simulink model "vC_3ph_MR2"  (Simulink 7.9)
settings: Solver=ode14x  StartTime=0.0  StopTime=20/60  FixedStep=Ts1  RelTol=1e-3
PostLoadFcn:
  | , if any(exist('dsrtsu_mdlpostloadfcn', 'file') == [2, 3, 6]), try dsrtsu_mdlpostloadfcn('Execute', bdroot); catch fprintf('Error in PostLoadFcn (dsrtsu_mdlpostloadfcn) for model "%s":\n %s\n', bdroot, lasterr); end, end,
InitFcn:
  | vC_ini
values from neighbouring files (symbols this model uses):
  C = Cideal+deltaC    (= 4e-05)    [IMC_calculo_limites_thetas.m]    (also in IMC_ini.m; JORGE_controlador_LCL_malha_interna.m; LCL_PAPM.m; R_in_LCL.m)
  excitacao_persistente = 0    [iC_ini.m]    (also in vC_ini.m)
  flag_time = 60/60    (= 1)    [iC_ini.m]    (also in vC_ini.m = 0)
  init_time = 60/60    (= 1)    [iC_ini.m]    (also in vC_ini.m)
  L1 = L1ideal+deltaL1    (= 0.002)    [IMC_calculo_limites_thetas.m]    (also in IMC_ini.m; LCL_PAPM.m; R_in_LCL.m; calculo_FTs.m)
  L2 = L2ideal+deltaL2+Lgideal+deltaLg    (= 0.002)    [IMC_calculo_limites_thetas.m]    (also in IMC_ini.m; LCL_PAPM.m; R_in_LCL.m; calculo_FTs.m)
  param_change_time = 60/60    (= 1)    [iC_ini.m]    (also in vC_ini.m)
  R1 = R1ideal+deltaR1    (= 1)    [IMC_calculo_limites_thetas.m]    (also in IMC_ini.m; R_in_LCL.m = 0; gera_resultados.m = 0; iC_ini.m = 0)
  R2 = R2ideal+deltaR2+Rgideal+deltaRg    (= 1)    [IMC_calculo_limites_thetas.m]    (also in IMC_ini.m; R_in_LCL.m = 0; gera_resultados.m = 0; iC_ini.m = 0)
  R_init = 10    [iC_ini.m]    (also in vC_ini.m)
  ref_phaseInv_time = 60/60    (= 1)    [iC_ini.m]    (also in vC_ini.m)
  ref_step_time = 60/60    (= 1)    [iC_ini.m]    (also in vC_ini.m)
  short_OFF_time = 61/60    (= 1.01666666667)    [vC_ini.m]
  short_ON_time = 60/60    (= 1)    [vC_ini.m]
  Ts = 0.5    [IMC_calculo_limites_thetas.m]    (also in IMC_datta_ini.m; IMC_ini.m = 8.33333333333e-05; JORGE_controlador_LCL_malha_interna.m = 8.33333333333e-05; LCL_PAPM.m = 8.33333333333e-05)
  Ts1 = Ts/10    (= 8.33333333333e-06)    [iC_ini.m]    (also in vC_ini.m)
  VCC = 1700    [iC_ini.m]    (also in vC_ini.m = 1200)
undefined symbols (not defined in the file or in its folder): D1, Delta
libraries: powerlib x38, powerlib_extras x1
(part 2 of 3)

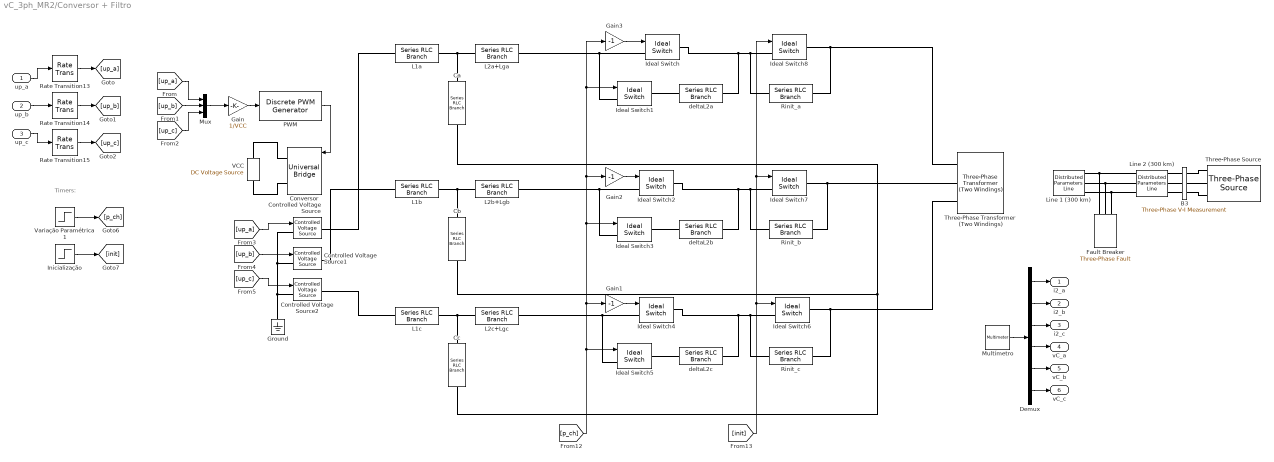
== system vC_3ph_MR2/Conversor + Filtro ==
  note: Timers:
  up_a : Inport
  up_b : Inport  Port=2
  up_c : Inport  Port=3
  B3 : powerlib/Measurements/Three-Phase V-I Measurement  VoltageMeasurement=no  SetLabelV=on  LabelV=Vabc_B3  Vpu=on  VpuLL=off  CurrentMeasurement=no  SetLabelI=on  LabelI=Iabc_B3  Ipu=on  Pbase=100e6  Vbase=735e3  OutputType=Complex  PhasorSimulation=off  PSBequivalent=0
  Ca : powerlib/Elements/Series RLC Branch  LConnTagsString=__new0  RConnTagsString=__new0  BranchType=C  Resistance=1  Inductance=1e-3  SetiL0=off  InitialCurrent=0  Capacitance=C  Setx0=off  InitialVoltage=0  Measurements=Branch voltage
  Cb : powerlib/Elements/Series RLC Branch  LConnTagsString=__new0  RConnTagsString=__new0  BranchType=C  Resistance=1  Inductance=1e-3  SetiL0=off  InitialCurrent=0  Capacitance=C  Setx0=off  InitialVoltage=0  Measurements=Branch voltage
  Cc : powerlib/Elements/Series RLC Branch  LConnTagsString=__new0  RConnTagsString=__new0  BranchType=C  Resistance=1  Inductance=1e-3  SetiL0=off  InitialCurrent=0  Capacitance=C  Setx0=off  InitialVoltage=0  Measurements=Branch voltage
  Controlled Voltage Source : powerlib/Electrical Sources/Controlled Voltage Source  Initialize=on  Source_Type=AC  Amplitude=0  Phase=0  Frequency=0  Measurements=None
  Controlled Voltage Source1 : powerlib/Electrical Sources/Controlled Voltage Source  Initialize=on  Source_Type=AC  Amplitude=0  Phase=0  Frequency=0  Measurements=None
  Controlled Voltage Source2 : powerlib/Electrical Sources/Controlled Voltage Source  Initialize=on  Source_Type=AC  Amplitude=0  Phase=0  Frequency=0  Measurements=None
  Conversor : powerlib/Power Electronics/Universal Bridge  Arms=3  SnubberResistance=1e5  SnubberCapacitance=inf  Device=IGBT / Diodes  Ron=1e-3  Lon=0  ForwardVoltages="[  0  0  ]"  ForwardVoltage=0  GTOparameters=[ 10e-6 , 20e-6 ]  IGBTparameters=[ 1e-6 , 2e-6 ]  Measurements=UAB UBC UCA UDC voltages  Measurements_2=None  converterType=Rectifier
  Demux : Demux  Outputs=6
  Fault Breaker : powerlib/Elements/Three-Phase Fault  FaultA=on  FaultB=off  FaultC=off  FaultResistance=0.001  GroundFault=on  GroundResistance=1  External=off  SwitchStatus=[1 0]  SwitchTimes=[ short_ON_time short_OFF_time ]  InitialStates=[0 0 1]  SnubberResistance=inf  SnubberCapacitance=inf  Measurements=Fault currents
  Gain : Gain  Gain=1/VCC  SampleTime=Ts1
  Gain1 : Gain  Gain=-1  SampleTime=Ts1
  Gain2 : Gain  Gain=-1  SampleTime=Ts1
  Gain3 : Gain  Gain=-1  SampleTime=Ts1
  Ground : powerlib/Elements/Ground  LConnTagsString=a
  Ideal Switch : powerlib/Power Electronics/Ideal Switch  Ron=0.001  Lon=0  IC=1  Rs=1e5  Cs=inf  Measurements=off
  Ideal Switch{1,3,5..8} (6 alike) : powerlib/Power Electronics/Ideal Switch  Ron=0.001  Lon=0  IC=0  Rs=1e5  Cs=inf  Measurements=off
  Ideal Switch2 : powerlib/Power Electronics/Ideal Switch  Ron=0.001  Lon=0  IC=1  Rs=1e5  Cs=inf  Measurements=off
  Ideal Switch4 : powerlib/Power Electronics/Ideal Switch  Ron=0.001  Lon=0  IC=1  Rs=1e5  Cs=inf  Measurements=off
  Inicialização : Step  Time=init_time  SampleTime=Ts1
  L1a : powerlib/Elements/Series RLC Branch  LConnTagsString=__new0  RConnTagsString=__new0  BranchType=RL  Resistance=R1  Inductance=L1  SetiL0=off  InitialCurrent=0  Capacitance=1e-6  Setx0=off  InitialVoltage=0  Measurements=None
  L1b : powerlib/Elements/Series RLC Branch  LConnTagsString=__new0  RConnTagsString=__new0  BranchType=RL  Resistance=R1  Inductance=L1  SetiL0=off  InitialCurrent=0  Capacitance=1e-6  Setx0=off  InitialVoltage=0  Measurements=None
  L1c : powerlib/Elements/Series RLC Branch  LConnTagsString=__new0  RConnTagsString=__new0  BranchType=RL  Resistance=R1  Inductance=L1  SetiL0=off  InitialCurrent=0  Capacitance=1e-6  Setx0=off  InitialVoltage=0  Measurements=None
  L2a+Lga : powerlib/Elements/Series RLC Branch  LConnTagsString=__new0  RConnTagsString=__new0  BranchType=RL  Resistance=R2  Inductance=L2  SetiL0=off  InitialCurrent=0  Capacitance=1e-6  Setx0=off  InitialVoltage=0  Measurements=Branch current
  L2b+Lgb : powerlib/Elements/Series RLC Branch  LConnTagsString=__new0  RConnTagsString=__new0  BranchType=RL  Resistance=R2  Inductance=L2  SetiL0=off  InitialCurrent=0  Capacitance=1e-6  Setx0=off  InitialVoltage=0  Measurements=Branch current
  L2c+Lgc : powerlib/Elements/Series RLC Branch  LConnTagsString=__new0  RConnTagsString=__new0  BranchType=RL  Resistance=R2  Inductance=L2  SetiL0=off  InitialCurrent=0  Capacitance=1e-6  Setx0=off  InitialVoltage=0  Measurements=Branch current
  Line 1 (300 km) : powerlib/Elements/Distributed Parameters Line  Phases=3  Frequency=60  Resistance=[0.01273 0.3864]  Inductance="[0.9337e-3  4.1264e-3]"  Capacitance=[12.74e-9 7.751e-9]  Length=300  x1=[-0.0017 3.92005703085229e-11 -7396.02996094138 -52768.9690973413;-0.00169166666666667 3.90926214322584e-11 -7230.2151300675 -52791.9439683011;-0.00168333333333333 3.89842867276027e-11 -7064.32893988924 -52814.3978040869;-0.001675 3.88755672637756e-11 -6898.37302763633 -52836.3303830885;-0.00166666666666667 3.87664641137943e-11 -6732.34903122663 -52857.74148884;-0.00165833333333333 3.86569783544628e-11 -6566.25858924993 -52878.6309100226;-0.00165 3.85471110663615e-11 -6400.10334095188 -52898.9984404661;-0.00164166666666667 3.8436863333836e-11 -6233.88492621767 -52918.8438791512;-0.00163333333333333 3.8326236244987e-11 -6067.60498555597 -52938.1670302113;-0.001625 3.82152308916592e-11 -5901.26516008265 -52956.9677029349;-0.00161666666666667 3.81038483694306e-11 -5734.86709150463 -52975.2457117669;-0.00160833333333333 3.79920897776017e-11 -5568.41242210368 -52993.0008763106;-0.0016 3.78799562191848e-11 -5401.90279472019 -53010.2330213299;-0.00159166666666667 3.77674488008927e-11 -5235.33985273694 -53026.9419767503;-0.00158333333333333 3.76545686331283e-11 -5068.72524006294 -53043.1275776612;-0.001575 3.75413168299733e-11 -4902.06060111715 -53058.7896643174;-0.00156666666666667 3.74276945091772e-11 -4735.34758081227 -53073.9280821402;-0.00155833333333333 3.73137027921465e-11 -4568.5878245385 -53088.5426817197;-0.00155 3.71993428039333e-11 -4401.78297814733 -53102.6333188156;-0.00154166666666667 3.70846156732247e-11 -4234.93468793522 -53116.1998543591;-0.00153333333333333 3.6969522532331e-11 -4068.04460062746 -53129.2421544539;-0.001525 3.68540645171751e-11 -3901.11436336182 -53141.7600903778;-0.00151666666666667 3.67382427672811e-11 -3734.14562367236 -53153.7535385837;-0.00150833333333333 3.66220584257627e-11 -3567.14002947314 -53165.2223807013;-0.0015 3.65055126393127e-11 -3400.09922904194 -53176.1665035377;-0.00149166666666667 3.63886065581907e-11 -3233.02487100401 -53186.5857990787;-0.00148333333333333 3.62713413362127e-11 -3065.91860431584 -53196.4801644903;-0.001475 3.6153718130739e-11 -2898.78207824881 -53205.8495021188;-0.00146666666666667 3.60357381026632e-11 -2731.61694237295 -53214.6937194929;-0.00145833333333333 3.59174024164006e-11 -2564.42484654066 -53223.0127293236;-0.00145 3.57987122398765e-11 -2397.20744087044 -53230.8064495056;-0.00144166666666667 3.56796687445152e-11 -2229.96637573058 -53238.0748031182;-0.00143333333333333 3.55602731052279e-11 -2062.70330172285 -53244.8177184255;-0.001425 3.54405265004012e-11 -1895.41986966628 -53251.0351288777;-0.00141666666666667 3.53204301118859e-11 -1728.11773058082 -53256.7269731115;-0.00140833333333333 3.51999851249848e-11 -1560.79853567102 -53261.8931949508;-0.0014 3.50791927284414e-11 -1393.46393630979 -53266.5337434068;-0.00139166666666667 3.49580541144278e-11 -1226.11558402208 -53270.6485726794;-0.00138333333333333 3.48365704785332e-11 -1058.75513046855 -53274.2376421568;-0.001375 3.47147430197521e-11 -891.384227429335 -53277.3009164164;-0.00136666666666667 3.45925729404722e-11 -724.004526787645 -53279.8383652248;-0.00135833333333333 3.44700614464631e-11 -556.617680513576 -53281.8499635386;-0.00135 3.43472097468636e-11 -389.225340647714 -53283.3356915039;-0.00134166666666667 3.42240190541704e-11 -221.82915928488 -53284.2955344573;-0.00133333333333333 3.41004905842259e-11 -54.4307885578019 -53284.7294829255;-0.001325 3.39766255562063e-11 112.968119379191 -53284.6375326256;-0.00131666666666667 3.38524251926094e-11 280.365912366451 -53284.0196844652;-0.00130833333333333 3.37278907192426e-11 447.760938255349 -53282.8759445421;-0.0013 3.3603023365211e-11 615.151544924549 -53281.2063241446;-0.00129166666666667 3.34778243629047e-11 782.536080296351 -53279.0108397512;-0.00128333333333333 3.33522949479876e-11 949.912892352961 -53276.2895130304;-0.001275 3.32264363593842e-11 1117.28032915281 -53273.0423708406;-0.00126666666666667 3.3100249839268e-11 1284.63673884689 -53269.2694452298;-0.00125833333333333 3.2973736633049e-11 1451.98046969498 -53264.9707734353;-0.00125 ...(+10984 chars)]  x2=[-0.0017 -3.86024177087245e-11 -6618.00740677682 -48900.0765944437;-0.00169166666666667 -3.86499120226598e-11 -6464.35087955851 -48920.6263316872;-0.00168333333333333 -3.8697024877567e-11 -6310.63055180679 -48940.6932420988;-0.001675 -3.87437558084613e-11 -6156.84794067921 -48960.2771276263;-0.00166666666666667 -3.87901043541273e-11 -6003.0045639481 -48979.3777949846;-0.00165833333333333 -3.88360700571234e-11 -5849.10193998543 -48997.9950556579;-0.00165 -3.88816524637869e-11 -5695.14158774801 -49016.1287259012;-0.00164166666666667 -3.89268511242377e-11 -5541.12502676233 -49033.7786267426;-0.00163333333333333 -3.89716655923833e-11 -5387.05377710968 -49050.9445839847;-0.001625 -3.9016095425923e-11 -5232.92935941109 -49067.6264282065;-0.00161666666666667 -3.90601401863523e-11 -5078.75329481235 -49083.8239947648;-0.00160833333333333 -3.91037994389672e-11 -4924.52710496895 -49099.5371237962;-0.0016 -3.91470727528684e-11 -4770.25231203115 -49114.7656602185;-0.00159166666666667 -3.91899597009659e-11 -4615.93043862886 -49129.5094537321;-0.00158333333333333 -3.92324598599828e-11 -4461.56300785665 -49143.7683588218;-0.001575 -3.92745728104597e-11 -4307.15154325877 -49157.542234758;-0.00156666666666667 -3.93162981367586e-11 -4152.69756881403 -49170.830945598;-0.00155833333333333 -3.93576354270677e-11 -3998.20260892079 -49183.6343601876;-0.00155 -3.93985842734043e-11 -3843.66818838195 -49195.9523521624;-0.00154166666666667 -3.94391442716201e-11 -3689.09583238984 -49207.7847999486;-0.00153333333333333 -3.94793150214041e-11 -3534.48706651121 -49219.1315867649;-0.001525 -3.95190961262872e-11 -3379.84341667215 -49229.9926006229;-0.00151666666666667 -3.95584871936462e-11 -3225.16640914308 -49240.367734329;-0.00150833333333333 -3.95974878347069e-11 -3070.4575705236 -49250.2568854846;-0.0015 -3.96360976645489e-11 -2915.7184277275 -49259.6599564879;-0.00149166666666667 -3.96743163021086e-11 -2760.95050796763 -49268.5768545344;-0.00148333333333333 -3.97121433701836e-11 -2606.15533874089 -49277.0074916179;-0.001475 -3.9749578495436e-11 -2451.33444781311 -49284.9517845313;-0.00146666666666667 -3.97866213083962e-11 -2296.48936320397 -49292.4096548678;-0.00145833333333333 -3.98232714434666e-11 -2141.62161317194 -49299.3810290211;-0.00145 -3.98595285389251e-11 -1986.73272619921 -49305.8658381866;-0.00144166666666667 -3.98953922369289e-11 -1831.82423097654 -49311.8640183619;-0.00143333333333333 -3.99308621835178e-11 -1676.89765638824 -49317.3755103474;-0.001425 -3.99659380286176e-11 -1521.95453149707 -49322.4002597467;-0.00141666666666667 -4.0000619426044e-11 -1366.99638552912 -49326.9382169678;-0.00140833333333333 -4.00349060335056e-11 -1212.02474785872 -49330.9893372228;-0.0014 -4.00687975126074e-11 -1057.04114799336 -49334.5535805287;-0.00139166666666667 -4.01022935288541e-11 -902.047115558624 -49337.630911708;-0.00138333333333333 -4.01353937516537e-11 -747.044180283028 -49340.2213003885;-0.001375 -4.01680978543202e-11 -592.033871982974 -49342.3247210043;-0.00136666666666667 -4.02004055140775e-11 -437.017720547603 -49343.9411527954;-0.00135833333333333 -4.02323164120619e-11 -281.997255923769 -49345.0705798083;-0.00135 -4.02638302333257e-11 -126.97400810086 -49345.7129908959;-0.00134166666666667 -4.02949466668403e-11 28.0504929042399 -49345.868379718;-0.00133333333333333 -4.0325665405499e-11 183.0747170623 -49345.536744741;-0.001325 -4.03559861461203e-11 338.097134346815 -49344.7180892378;-0.00131666666666667 -4.03859085894508e-11 493.116214749112 -49343.4124212884;-0.00130833333333333 -4.04154324401678e-11 648.130428293447 -49341.6197537792;-0.0013 -4.04445574068831e-11 803.138245052112 -49339.3401044029;-0.00129166666666667 -4.04732832021449e-11 958.138135160545 -49336.573495659;-0.00128333333333333 -4.05016095424412e-11 1113.1285688324 -49333.3199548526;-0.001275 -4.05295361482025e-11 1268.10801637466 -49329.5795140949;-0.00126666666666667 -4.05570627438045e-11 1423.07494820276 -49325.3522103026;-0.00125833333333333 -4.05841890575707e-11 ...(+11172 chars)]  x3=[-0.0017 -2.15563861094982e-14 -27.7294039862374 -193.67611553396;-0.00169166666666667 -2.22240906952308e-14 -27.1208166863509 -193.762274129979;-0.00168333333333333 -2.28915759381605e-14 -26.5119617149528 -193.846520370577;-0.001675 -2.35588352504773e-14 -25.9028450811959 -193.928853424279;-0.00166666666666667 -2.42258620466013e-14 -25.2934727968154 -194.009272478489;-0.00165833333333333 -2.48926497432473e-14 -24.6838508760698 -194.087776739504;-0.00165 -2.55591917594899e-14 -24.0739853356814 -194.16436543252;-0.00164166666666667 -2.62254815168285e-14 -23.4638821947767 -194.239037801636;-0.00163333333333333 -2.68915124392521e-14 -22.8535474748276 -194.311793109867;-0.001625 -2.75572779533045e-14 -22.2429871995912 -194.382630639146;-0.00161666666666667 -2.82227714881489e-14 -21.632207395051 -194.451549690336;-0.00160833333333333 -2.88879864756327e-14 -21.021214089357 -194.518549583234;-0.0016 -2.95529163503525e-14 -20.4100133127667 -194.583629656578;-0.00159166666666667 -3.02175545497189e-14 -19.7986110975848 -194.646789268054;-0.00158333333333333 -3.08818945140212e-14 -19.1870134781044 -194.708027794302;-0.001575 -3.15459296864923e-14 -18.575226490547 -194.767344630923;-0.00156666666666667 -3.22096535133728e-14 -17.9632561730033 -194.824739192482;-0.00155833333333333 -3.28730594439768e-14 -17.3511085653733 -194.88021091252;-0.00155 -3.35361409307555e-14 -16.7387897093067 -194.933759243553;-0.00154166666666667 -3.41988914293622e-14 -16.1263056481433 -194.985383657079;-0.00153333333333333 -3.48613043987172e-14 -15.5136624268536 -195.035083643588;-0.001525 -3.5523373301072e-14 -14.9008660919789 -195.08285871256;-0.00151666666666667 -3.61850916020735e-14 -14.2879226915716 -195.128708392475;-0.00150833333333333 -3.68464527708295e-14 -13.6748382751356 -195.172632230814;-0.0015 -3.75074502799721e-14 -13.0616188935666 -195.214629794068;-0.00149166666666667 -3.81680776057228e-14 -12.4482705990923 -195.254700667737;-0.00148333333333333 -3.88283282279567e-14 -11.8347994452128 -195.292844456338;-0.001475 -3.94881956302665e-14 -11.2212114866406 -195.329060783407;-0.00146666666666667 -4.01476733000276e-14 -10.6075127792412 -195.363349291503;-0.00145833333333333 -4.08067547284614e-14 -9.99370937997315 -195.395709642214;-0.00145 -4.14654334107004e-14 -9.37980734682814 -195.426141516155;-0.00144166666666667 -4.21237028458519e-14 -8.7658127387714 -195.454644612975;-0.00143333333333333 -4.27815565370624e-14 -8.15173161568181 -195.481218651362;-0.001425 -4.34389879915814e-14 -7.53757003829216 -195.50586336904;-0.00141666666666667 -4.4095990720826e-14 -6.92333406812929 -195.528578522775;-0.00140833333333333 -4.47525582404444e-14 -6.30902976745423 -195.549363888378;-0.0014 -4.54086840703804e-14 -5.69466319920241 -195.568219260705;-0.00139166666666667 -4.60643617349368e-14 -5.08024042692384 -195.585144453663;-0.00138333333333333 -4.67195847628398e-14 -4.46576751472323 -195.600139300206;-0.001375 -4.73743466873027e-14 -3.85125052720019 -195.613203652342;-0.00136666666666667 -4.80286410460896e-14 -3.23669552938921 -195.624337381129;-0.00135833333333333 -4.86824613815793e-14 -2.62210858670008 -195.633540376683;-0.00135 -4.9335801240829e-14 -2.00749576485779 -195.640812548174;-0.00134166666666667 -4.99886541756382e-14 -1.39286312984277 -195.646153823829;-0.00133333333333333 -5.06410137426119e-14 -0.778216747830982 -195.649564150931;-0.001325 -5.12928735032246e-14 -0.163562685134053 -195.651043495821;-0.00131666666666667 -5.19442270238835e-14 0.451092991860548 -195.6505918439;-0.00130833333333333 -5.25950678759925e-14 1.06574421674942 -195.648209199625;-0.0013 -5.3245389636015e-14 1.68038492317314 -195.643895586511;-0.00129166666666667 -5.38951858855379e-14 2.29500904487608 -195.637651047133;-0.00128333333333333 -5.45444502113344e-14 2.90961051576626 -195.62947564312;-0.001275 -5.51931762054278e-14 3.52418326997528 -195.619369455162;-0.00126666666666667 -5.58413574651545e-14 4.13872124191825 -195.607332583003;-0.00125833333333333 -5.6488987593227e-14 ...(+11158 chars)]  x4=[-0.0017 -1.25069855625768e-15 -97.1520132574429 -167.719905551199;-0.00169166666666667 -1.17646120080317e-15 -96.6246270754558 -168.024289436398;-0.00168333333333333 -1.10221223415156e-15 -96.0962872474085 -168.327014989695;-0.001675 -1.02795238911018e-15 -95.5669989878017 -168.62807922331;-0.00166666666666667 -9.53682398593721e-16 -95.0367675204968 -168.927479165861;-0.00165833333333333 -8.79402995617002e-16 -94.5055980786644 -169.225211862392;-0.00165 -8.05114913287751e-16 -93.9734959047324 -169.5212743744;-0.00164166666666667 -7.30818884799338e-16 -93.4404662503344 -169.815663779869;-0.00163333333333333 -6.56515643423579e-16 -92.906514376258 -170.108377173294;-0.001625 -5.82205922503465e-16 -92.3716455523927 -170.399411665711;-0.00161666666666667 -5.07890455445944e-16 -91.8358650576776 -170.688764384729;-0.00160833333333333 -4.33569975714665e-16 -91.29917818005 -170.976432474552;-0.0016 -3.59245216822771e-16 -90.7615902163928 -171.262413096012;-0.00159166666666667 -2.84916912325618e-16 -90.2231064724821 -171.546703426596;-0.00158333333333333 -2.10585795813567e-16 -89.6837322629351 -171.829300660474;-0.001575 -1.36252600904725e-16 -89.1434729111574 -172.110202008525;-0.00156666666666667 -6.19180612377231e-17 -88.6023337492907 -172.389404698365;-0.00155833333333333 1.24170895355471e-17 -88.0603201181601 -172.666905974378;-0.00155 8.67521177571522e-17 -87.5174373672214 -172.942703097737;-0.00154166666666667 1.61086289770384e-16 -86.9736908545081 -173.216793346436;-0.00153333333333333 2.35418871926968e-16 -86.4290859465787 -173.489174015315;-0.001525 3.09749130594331e-16 -85.8836280184639 -173.759842416088;-0.00151666666666667 3.84076332162822e-16 -85.3373224536132 -174.028795877365;-0.00150833333333333 4.58399743052972e-16 -84.7901746438419 -174.296031744685;-0.0015 5.32718629722723e-16 -84.2421899892781 -174.561547380538;-0.00149166666666667 6.07032258674666e-16 -83.693373898309 -174.825340164392;-0.00148333333333333 6.81339896463284e-16 -83.1437317875279 -175.087407492718;-0.001475 7.55640809702191e-16 -82.5932690816805 -175.347746779018;-0.00146666666666667 8.29934265071373e-16 -82.0419912136116 -175.606355453848;-0.00145833333333333 9.0421952932442e-16 -81.4899036242111 -175.863230964844;-0.00145 9.78495869295754e-16 -80.9370117623606 -176.11837077675;-0.00144166666666667 1.05276255190789e-15 -80.3833210848796 -176.371772371439;-0.00143333333333333 1.12701884417867e-15 -79.8288370564716 -176.623433247938;-0.001425 1.20126401322844e-15 -79.27356514967 -176.873350922457;-0.00141666666666667 1.27549732628738e-15 -78.7175108447845 -177.121522928408;-0.00140833333333333 1.34971805070264e-15 -78.1606796298464 -177.367946816436;-0.0014 1.42392545394565e-15 -77.6030770005551 -177.612620154434;-0.00139166666666667 1.49811880361929e-15 -77.0447084602235 -177.855540527577;-0.00138333333333333 1.57229736746515e-15 -76.4855795197236 -178.096705538338;-0.001375 1.64646041337075e-15 -75.9256956974323 -178.336112806516;-0.00136666666666667 1.72060720937678e-15 -75.3650625191769 -178.573759969258;-0.00135833333333333 1.79473702368429e-15 -74.8036855181805 -178.809644681081;-0.00135 1.86884912466194e-15 -74.2415702350076 -179.043764613901;-0.00134166666666667 1.94294278085322e-15 -73.6787222175089 -179.276117457046;-0.00133333333333333 2.01701726098364e-15 -73.1151470207673 -179.506700917289;-0.001325 2.09107183396801e-15 -72.5508502070424 -179.735512718863;-0.00131666666666667 2.16510576891757e-15 -71.9858373457159 -179.96255060349;-0.00130833333333333 2.23911833514728e-15 -71.4201140132366 -180.187812330395;-0.0013 2.31310880218299e-15 -70.8536857930655 -180.411295676338;-0.00129166666666667 2.38707643976867e-15 -70.2865582756204 -180.632998435627;-0.00128333333333333 2.46102051787358e-15 -69.718737058221 -180.852918420146;-0.001275 2.53494030669954e-15 -69.1502277450334 -181.071053459374;-0.00126666666666667 2.60883507668807e-15 -68.581035947015 -181.287401400405;-0.00125833333333333 2.68270409852762e-15 -68.0111672818591 ...(+11113 chars)]  x5=0.00169662470098723  Measurements=None
      settings: AttributesFormatString=\n
  Line 2 (300 km) : powerlib/Elements/Distributed Parameters Line  Phases=3  Frequency=60  Resistance=[0.01273 0.3864]  Inductance="[0.9337e-3  4.1264e-3]"  Capacitance=[12.74e-9 7.751e-9]  Length=300  x1=[-0.0017 -3.86024177087245e-11 -6618.00740677682 -48900.0765944437;-0.00169166666666667 -3.86499120226598e-11 -6464.35087955851 -48920.6263316872;-0.00168333333333333 -3.8697024877567e-11 -6310.63055180679 -48940.6932420988;-0.001675 -3.87437558084613e-11 -6156.84794067921 -48960.2771276263;-0.00166666666666667 -3.87901043541273e-11 -6003.0045639481 -48979.3777949846;-0.00165833333333333 -3.88360700571234e-11 -5849.10193998543 -48997.9950556579;-0.00165 -3.88816524637869e-11 -5695.14158774801 -49016.1287259012;-0.00164166666666667 -3.89268511242377e-11 -5541.12502676233 -49033.7786267426;-0.00163333333333333 -3.89716655923833e-11 -5387.05377710968 -49050.9445839847;-0.001625 -3.9016095425923e-11 -5232.92935941109 -49067.6264282065;-0.00161666666666667 -3.90601401863523e-11 -5078.75329481235 -49083.8239947648;-0.00160833333333333 -3.91037994389672e-11 -4924.52710496895 -49099.5371237962;-0.0016 -3.91470727528684e-11 -4770.25231203115 -49114.7656602185;-0.00159166666666667 -3.91899597009659e-11 -4615.93043862886 -49129.5094537321;-0.00158333333333333 -3.92324598599828e-11 -4461.56300785665 -49143.7683588218;-0.001575 -3.92745728104597e-11 -4307.15154325877 -49157.542234758;-0.00156666666666667 -3.93162981367586e-11 -4152.69756881403 -49170.830945598;-0.00155833333333333 -3.93576354270677e-11 -3998.20260892079 -49183.6343601876;-0.00155 -3.93985842734043e-11 -3843.66818838195 -49195.9523521624;-0.00154166666666667 -3.94391442716201e-11 -3689.09583238984 -49207.7847999486;-0.00153333333333333 -3.94793150214041e-11 -3534.48706651121 -49219.1315867649;-0.001525 -3.95190961262872e-11 -3379.84341667215 -49229.9926006229;-0.00151666666666667 -3.95584871936462e-11 -3225.16640914308 -49240.367734329;-0.00150833333333333 -3.95974878347069e-11 -3070.4575705236 -49250.2568854846;-0.0015 -3.96360976645489e-11 -2915.7184277275 -49259.6599564879;-0.00149166666666667 -3.96743163021086e-11 -2760.95050796763 -49268.5768545344;-0.00148333333333333 -3.97121433701836e-11 -2606.15533874089 -49277.0074916179;-0.001475 -3.9749578495436e-11 -2451.33444781311 -49284.9517845313;-0.00146666666666667 -3.97866213083962e-11 -2296.48936320397 -49292.4096548678;-0.00145833333333333 -3.98232714434666e-11 -2141.62161317194 -49299.3810290211;-0.00145 -3.98595285389251e-11 -1986.73272619921 -49305.8658381866;-0.00144166666666667 -3.98953922369289e-11 -1831.82423097654 -49311.8640183619;-0.00143333333333333 -3.99308621835178e-11 -1676.89765638824 -49317.3755103474;-0.001425 -3.99659380286176e-11 -1521.95453149707 -49322.4002597467;-0.00141666666666667 -4.0000619426044e-11 -1366.99638552912 -49326.9382169678;-0.00140833333333333 -4.00349060335056e-11 -1212.02474785872 -49330.9893372228;-0.0014 -4.00687975126074e-11 -1057.04114799336 -49334.5535805287;-0.00139166666666667 -4.01022935288541e-11 -902.047115558624 -49337.630911708;-0.00138333333333333 -4.01353937516537e-11 -747.044180283028 -49340.2213003885;-0.001375 -4.01680978543202e-11 -592.033871982974 -49342.3247210043;-0.00136666666666667 -4.02004055140775e-11 -437.017720547603 -49343.9411527954;-0.00135833333333333 -4.02323164120619e-11 -281.997255923769 -49345.0705798083;-0.00135 -4.02638302333257e-11 -126.97400810086 -49345.7129908959;-0.00134166666666667 -4.02949466668403e-11 28.0504929042399 -49345.868379718;-0.00133333333333333 -4.0325665405499e-11 183.0747170623 -49345.536744741;-0.001325 -4.03559861461203e-11 338.097134346815 -49344.7180892378;-0.00131666666666667 -4.03859085894508e-11 493.116214749112 -49343.4124212884;-0.00130833333333333 -4.04154324401678e-11 648.130428293447 -49341.6197537792;-0.0013 -4.04445574068831e-11 803.138245052112 -49339.3401044029;-0.00129166666666667 -4.04732832021449e-11 958.138135160545 -49336.573495659;-0.00128333333333333 -4.05016095424412e-11 1113.1285688324 -49333.3199548526;-0.001275 -4.05295361482025e-11 1268.10801637466 -49329.5795140949;-0.00126666666666667 -4.05570627438045e-11 1423.07494820276 -49325.3522103026;-0.00125833333333333 -4.05841890575707e-11 ...(+11172 chars)]  x2=[-0.0017 -1.78193727615485e-11 -4583.41557044112 -37720.1439036556;-0.00169166666666667 -1.78111380205216e-11 -4464.89182015718 -37734.3569633582;-0.00168333333333333 -1.78027274907531e-11 -4346.32400319353 -37748.1976001916;-0.001675 -1.77941412552516e-11 -4227.71328976664 -37761.6656775542;-0.00166666666666667 -1.77853793987596e-11 -4109.06085051638 -37774.7610625216;-0.00165833333333333 -1.77764420077532e-11 -3990.36785649442 -37787.4836258476;-0.00165 -1.77673291704408e-11 -3871.6354791527 -37799.8332419657;-0.00164166666666667 -1.77580409767625e-11 -3752.86489033183 -37811.80978899;-0.00163333333333333 -1.77485775183889e-11 -3634.05726224959 -37823.413148717;-0.001625 -1.77389388887206e-11 -3515.21376748931 -37834.6432066261;-0.00161666666666667 -1.7729125182887e-11 -3396.33557898829 -37845.4998518813;-0.00160833333333333 -1.77191364977454e-11 -3277.42387002625 -37855.9829773317;-0.0016 -1.77089729318801e-11 -3158.47981421378 -37866.0924795133;-0.00159166666666667 -1.76986345856013e-11 -3039.50458548066 -37875.8282586492;-0.00158333333333333 -1.76881215609444e-11 -2920.49935806438 -37885.1902186513;-0.001575 -1.76774339616686e-11 -2801.46530649849 -37894.1782671208;-0.00156666666666667 -1.76665718932563e-11 -2682.40360560103 -37902.7923153493;-0.00155833333333333 -1.76555354629118e-11 -2563.31543046291 -37911.0322783197;-0.00155 -1.764432477956e-11 -2444.20195643635 -37918.8980747068;-0.00154166666666667 -1.7632939953846e-11 -2325.06435912323 -37926.3896268783;-0.00153333333333333 -1.76213810981333e-11 -2205.90381436356 -37933.5068608957;-0.001525 -1.76096483265032e-11 -2086.72149822379 -37940.2497065148;-0.00151666666666667 -1.75977417547534e-11 -1967.51858698529 -37946.6180971864;-0.00150833333333333 -1.75856615003971e-11 -1848.29625713265 -37952.611970057;-0.0015 -1.75734076826613e-11 -1729.05568534215 -37958.2312659696;-0.00149166666666667 -1.75609804224863e-11 -1609.79804847006 -37963.475929464;-0.00148333333333333 -1.75483798425243e-11 -1490.52452354115 -37968.3459087773;-0.001475 -1.75356060671378e-11 -1371.23628773695 -37972.8411558451;-0.00146666666666667 -1.75226592223988e-11 -1251.93451838416 -37976.9616263008;-0.00145833333333333 -1.75095394360874e-11 -1132.62039294311 -37980.7072794773;-0.00145 -1.74962468376908e-11 -1013.29508899604 -37984.0780784063;-0.00144166666666667 -1.74827815584013e-11 -893.959784235527 -37987.0739898194;-0.00143333333333333 -1.7469143731116e-11 -774.615656452846 -37989.6949841483;-0.001425 -1.74553334904346e-11 -655.263883526362 -37991.9410355248;-0.00141666666666667 -1.74413509726586e-11 -535.905643409889 -37993.8121217812;-0.00140833333333333 -1.74271963157899e-11 -416.542114121072 -37995.3082244507;-0.0014 -1.74128696595293e-11 -297.174473729749 -37996.4293287673;-0.00139166666666667 -1.73983711452749e-11 -177.803900346342 -37997.1754236663;-0.00138333333333333 -1.73837009161214e-11 -58.431572110223 -37997.5465017839;-0.001375 -1.73688591168578e-11 60.9413328219143 -37997.5425594577;-0.00136666666666667 -1.73538458939669e-11 180.313636287712 -37997.1635967267;-0.00135833333333333 -1.73386613956231e-11 299.684160130708 -37996.4096173311;-0.00135 -1.73233057716912e-11 419.051726212034 -37995.2806287124;-0.00134166666666667 -1.7307779173725e-11 538.415156422001 -37993.7766420131;-0.00133333333333333 -1.72920817549658e-11 657.773272691735 -37991.8976720771;-0.001325 -1.72762136703408e-11 777.124897004825 -37989.6437374491;-0.00131666666666667 -1.72601750764615e-11 896.468851408923 -37987.0148603743;-0.00130833333333333 -1.72439661316225e-11 1015.80395802737 -37984.0110667989;-0.0013 -1.72275869957994e-11 1135.12903907085 -37980.632386369;-0.00129166666666667 -1.72110378306477e-11 1254.442916849 -37976.8788524309;-0.00128333333333333 -1.7194318799501e-11 1373.74441378198 -37972.7505020304;-0.001275 -1.71774300673693e-11 1493.0323524122 -37968.2473759126;-0.00126666666666667 -1.71603718009378e-11 1612.30555541587 -37963.3695185217;-0.00125833333333333 -1.71431441685644e-11 ...(+11173 chars)]  x3=[-0.0017 -8.13204885553383e-14 48.7742194936725 -189.740833778909;-0.00169166666666667 -8.1253444740059e-14 49.370066231705 -189.586668968601;-0.00168333333333333 -8.11855989860835e-14 49.9654257071152 -189.430633014408;-0.001675 -8.1116951963022e-14 50.5602920439456 -189.272727456344;-0.00166666666666667 -8.10475043483928e-14 51.1546593711055 -189.112953852873;-0.00165833333333333 -8.09772568276159e-14 51.7485218224294 -188.951313780895;-0.00165 -8.09062100940059e-14 52.3418735367347 -188.787808835733;-0.00164166666666667 -8.08343648487655e-14 52.9347086578794 -188.622440631114;-0.00163333333333333 -8.07617218009782e-14 53.5270213348202 -188.455210799156;-0.001625 -8.06882816676015e-14 54.1188057216702 -188.28612099035;-0.00161666666666667 -8.061404517346e-14 54.7100559777564 -188.115172873544;-0.00160833333333333 -8.05390130512378e-14 55.3007662676775 -187.942368135927;-0.0016 -8.04631860414717e-14 55.8909307613612 -187.767708483012;-0.00159166666666667 -8.03865648925436e-14 56.4805436341225 -187.591195638619;-0.00158333333333333 -8.03091503606735e-14 57.0695990667202 -187.412831344859;-0.001575 -8.02309432099114e-14 57.6580912454151 -187.232617362115;-0.00156666666666667 -8.01519442121303e-14 58.2460143620268 -187.050555469026;-0.00155833333333333 -8.00721541470186e-14 58.8333626139917 -186.866647462471;-0.00155 -7.99915738020718e-14 59.4201302044195 -186.680895157546;-0.00154166666666667 -7.99102039725856e-14 60.0063113421512 -186.493300387551;-0.00153333333333333 -7.98280454616471e-14 60.5919002418154 -186.303865003973;-0.001525 -7.97450990801279e-14 61.1768911238861 -186.112590876461;-0.00151666666666667 -7.96613656466751e-14 61.7612782147396 -185.919479892813;-0.00150833333333333 -7.9576845987704e-14 62.3450557467112 -185.724533958958;-0.0015 -7.94915409373894e-14 62.9282179581522 -185.527754998933;-0.00149166666666667 -7.94054513376579e-14 63.5107590934871 -185.329144954866;-0.00148333333333333 -7.93185780381789e-14 64.0926734032701 -185.128705786959;-0.001475 -7.92309218963569e-14 64.6739551442419 -184.926439473465;-0.00146666666666667 -7.91424837773226e-14 65.2545985793864 -184.722348010672;-0.00145833333333333 -7.90532645539245e-14 65.8345979779872 -184.516433412879;-0.00145 -7.89632651067203e-14 66.4139476156844 -184.308697712381;-0.00144166666666667 -7.88724863239684e-14 66.9926417745311 -184.099142959445;-0.00143333333333333 -7.87809291016185e-14 67.5706747430496 -183.887771222291;-0.001425 -7.86885943433035e-14 68.1480408162876 -183.674584587074;-0.00141666666666667 -7.85954829603302e-14 68.7247342958753 -183.45958515786;-0.00140833333333333 -7.85015958716704e-14 69.3007494900808 -183.242775056606;-0.0014 -7.84069340039517e-14 69.8760807138667 -183.02415642314;-0.00139166666666667 -7.83114982914486e-14 70.450722288946 -182.80373141514;-0.00138333333333333 -7.82152896760729e-14 71.0246685438385 -182.581502208111;-0.001375 -7.8118309107365e-14 71.5979138139262 -182.357470995368;-0.00136666666666667 -7.80205575424837e-14 72.1704524415099 -182.131639988006;-0.00135833333333333 -7.79220359461978e-14 72.7422787758643 -181.904011414887;-0.00135 -7.78227452908754e-14 73.3133871732945 -181.674587522612;-0.00134166666666667 -7.77226865564753e-14 73.8837719971911 -181.443370575504;-0.00133333333333333 -7.76218607305368e-14 74.4534276180861 -181.21036285558;-0.001325 -7.75202688081701e-14 75.0223484137087 -180.975566662533;-0.00131666666666667 -7.74179117920465e-14 75.5905287690401 -180.738984313705;-0.00130833333333333 -7.73147906923884e-14 76.1579630763697 -180.500618144069;-0.0013 -7.72109065269594e-14 76.72464573535 -180.260470506203;-0.00129166666666667 -7.71062603210542e-14 77.2905711530518 -180.018543770268;-0.00128333333333333 -7.70008531074888e-14 77.8557337440199 -179.774840323981;-0.001275 -7.68946859265897e-14 78.4201279303275 -179.529362572599;-0.00126666666666667 -7.67877598261841e-14 78.9837481416319 -179.282112938887;-0.00125833333333333 -7.66800758615895e-14 79.5465888152292 -179.0330938631;-0.00125 ...(+11126 chars)]  x4=[-0.0017 4.97585139957785e-14 -152.47288977289 -118.697101129343;-0.00169166666666667 4.96176644384028e-14 -152.099240022438 -119.175522305555;-0.00168333333333333 4.94763251747106e-14 -151.724089113893 -119.652767267476;-0.001675 4.93344975996632e-14 -151.347440749842 -120.128831304889;-0.00166666666666667 4.91921831130417e-14 -150.969298647652 -120.603709719235;-0.00165833333333333 4.90493831194326e-14 -150.589666539433 -121.077397823656;-0.00165 4.89060990282141e-14 -150.208548172 -121.549890943041;-0.00164166666666667 4.87623322535424e-14 -149.825947306839 -122.021184414074;-0.00163333333333333 4.86180842143374e-14 -149.441867720065 -122.491273585279;-0.001625 4.84733563342693e-14 -149.056313202389 -122.960153817066;-0.00161666666666667 4.83281500417435e-14 -148.669287559078 -123.427820481775;-0.00160833333333333 4.81824667698878e-14 -148.280794609919 -123.894268963726;-0.0016 4.8036307956537e-14 -147.890838189181 -124.359494659261;-0.00159166666666667 4.78896750442198e-14 -147.499422145576 -124.823492976789;-0.00158333333333333 4.77425694801437e-14 -147.106550342222 -125.286259336835;-0.001575 4.75949927161814e-14 -146.712226656605 -125.747789172081;-0.00156666666666667 4.74469462088557e-14 -146.316454980542 -126.208077927415;-0.00155833333333333 4.72984314193261e-14 -145.919239220138 -126.667121059972;-0.00155 4.71494498133736e-14 -145.520583295753 -127.124914039181;-0.00154166666666667 4.70000028613864e-14 -145.12049114196 -127.581452346811;-0.00153333333333333 4.68500920383456e-14 -144.718966707507 -128.036731477013;-0.001525 4.66997188238106e-14 -144.316013955278 -128.490746936367;-0.00151666666666667 4.65488847019042e-14 -143.911636862254 -128.943494243921;-0.00150833333333333 4.63975911612983e-14 -143.505839419473 -129.394968931244;-0.0015 4.62458396951991e-14 -143.098625631993 -129.845166542463;-0.00149166666666667 4.60936318013324e-14 -142.68999951885 -130.294082634308;-0.00148333333333333 4.59409689819285e-14 -142.279965113017 -130.74171277616;-0.001475 4.57878527437079e-14 -141.86852646137 -131.188052550089;-0.00146666666666667 4.5634284597866e-14 -141.455687624641 -131.633097550903;-0.00145833333333333 4.54802660600584e-14 -141.041452677383 -132.076843386185;-0.00145 4.5325798650386e-14 -140.625825707928 -132.519285676346;-0.00144166666666667 4.51708838933796e-14 -140.208810818346 -132.960420054656;-0.00143333333333333 4.50155233179855e-14 -139.790412124406 -133.4002421673;-0.001425 4.48597184575496e-14 -139.370633755533 -133.838747673408;-0.00141666666666667 4.47034708498033e-14 -138.949479854772 -134.275932245111;-0.00140833333333333 4.45467820368471e-14 -138.526954578741 -134.711791567571;-0.0014 4.43896535651365e-14 -138.103062097594 -135.146321339034;-0.00139166666666667 4.4232086985466e-14 -137.677806594979 -135.579517270866;-0.00138333333333333 4.40740838529543e-14 -137.251192267995 -136.011375087598;-0.001375 4.39156457270283e-14 -136.823223327154 -136.441890526968;-0.00136666666666667 4.37567741714084e-14 -136.393903996336 -136.871059339963;-0.00135833333333333 4.35974707540928e-14 -135.963238512751 -137.298877290858;-0.00135 4.34377370473419e-14 -135.531231126892 -137.725340157265;-0.00134166666666667 4.32775746276628e-14 -135.097886102498 -138.150443730167;-0.00133333333333333 4.31169850757941e-14 -134.663207716509 -138.574183813962;-0.001325 4.29559699766896e-14 -134.227200259026 -138.996556226508;-0.00131666666666667 4.27945309195035e-14 -133.789868033266 -139.417556799159;-0.00130833333333333 4.26326694975741e-14 -133.351215355522 -139.837181376809;-0.0013 4.24703873084083e-14 -132.911246555118 -140.255425817934;-0.00129166666666667 4.23076859536657e-14 -132.469965974369 -140.67228599463;-0.00128333333333333 4.2144567039143e-14 -132.027377968536 -141.087757792654;-0.001275 4.19810321747582e-14 -131.583486905784 -141.501837111469;-0.00126666666666667 4.18170829745342e-14 -131.138297167139 -141.914519864277;-0.00125833333333333 4.16527210565834e-14 -130.691813146444 -142.325801978068;-0.00125 ...(+11131 chars)]  x5=0.00169662470098723  Measurements=None
      settings: AttributesFormatString=\n
  Multímetro : powerlib/Measurements/Multimeter  PhasorSimulation=off  OutputType=Complex  sel=[8 9 10 1 2 3]  L=13  Gain=[1 1 1 1 1 1]  yselected={'Ib: Conversor + Filtro/L2a+Lga','Ib: Conversor + Filtro/L2b+Lgb','Ib: Conversor + Filtro/L2c+Lgc','Ub: Conversor + Filtro/Ca','Ub: Conversor + Filtro/Cb','Ub: Conversor + Filtro/Cc'};  PSBOutputType=1  PSBequivalent=0  AxesSetting=[0,0.1,-100,100]  Display=0  SavedBlockNames=-11
  Mux : Mux  Inputs=3
  PWM : powerlib_extras/Discrete  Control Blocks/Discrete PWM Generator  GeneratorMode="3-arm  bridge (6 pulses)"  Fc=12000  Ts=Ts1  Internal=off  mIndex=0.4  Freq=60  Phase=0
  Rate Transition13 : RateTransition  OutPortSampleTime=Ts1
  Rate Transition14 : RateTransition  OutPortSampleTime=Ts1
  Rate Transition15 : RateTransition  OutPortSampleTime=Ts1
  Rinit_a : powerlib/Elements/Series RLC Branch  LConnTagsString=__new0  RConnTagsString=__new0  BranchType=RL  Resistance=R_init  Inductance=5*L2  SetiL0=off  InitialCurrent=0  Capacitance=1e-6  Setx0=off  InitialVoltage=0  Measurements=None
  Rinit_b : powerlib/Elements/Series RLC Branch  LConnTagsString=__new0  RConnTagsString=__new0  BranchType=RL  Resistance=R_init  Inductance=5*L2  SetiL0=off  InitialCurrent=0  Capacitance=1e-6  Setx0=off  InitialVoltage=0  Measurements=None
  Rinit_c : powerlib/Elements/Series RLC Branch  LConnTagsString=__new0  RConnTagsString=__new0  BranchType=RL  Resistance=R_init  Inductance=5*L2  SetiL0=off  InitialCurrent=0  Capacitance=1e-6  Setx0=off  InitialVoltage=0  Measurements=None
  Three-Phase Transformer (Two Windings) : powerlib/Elements/Three-Phase Transformer (Two Windings)  Winding1Connection=Yg  UNITS=pu  NominalPower=[ 2.5e6 , 60 ]  Winding1=[ 440 , 0.002 , 0.08 ]  Winding2Connection=Delta (D1)  Winding2=[ 34.5e3 , 0.002 , 0.08 ]  SetSaturation=off  Rm=500  Lm=500  Saturation=[ 0,0 ; 0.0024,1.2 ; 1.0,1.52 ]  Hysteresis=off  DataFile='hysteresis'  SetInitialFlux=off  InitialFluxes=[ 0.8 , -0.8 , 0.7 ]  Measurements=None  MoreParameters=off  BreakLoop=off  DataType=off  TransfoNumber=1
  Three-Phase Source : powerlib/Electrical Sources/Three-Phase Source  Voltage=38e3  PhaseAngle=0  Frequency=60  InternalConnection=Yg  SpecifyImpedance=off  Resistance=1  Inductance=0.01e-3  ShortCircuitLevel=100e6  BaseVoltage=380e3  XRratio=7  BusType=swing  Pref=0  Qref=0  Qmin=-inf  Qmax=inf
  VCC : powerlib/Electrical Sources/DC Voltage Source  Amplitude=VCC  Measurements=None
  Variação Paramétrica1 : Step  Time=param_change_time  Before=-1  SampleTime=Ts1
  deltaL2a : powerlib/Elements/Series RLC Branch  LConnTagsString=__new0  RConnTagsString=__new0  BranchType=RL  Resistance=0  Inductance=5*L2  SetiL0=off  InitialCurrent=0  Capacitance=1e-6  Setx0=off  InitialVoltage=0  Measurements=None
  deltaL2b : powerlib/Elements/Series RLC Branch  LConnTagsString=__new0  RConnTagsString=__new0  BranchType=RL  Resistance=0  Inductance=5*L2  SetiL0=off  InitialCurrent=0  Capacitance=1e-6  Setx0=off  InitialVoltage=0  Measurements=None
  deltaL2c : powerlib/Elements/Series RLC Branch  LConnTagsString=__new0  RConnTagsString=__new0  BranchType=RL  Resistance=0  Inductance=5*L2  SetiL0=off  InitialCurrent=0  Capacitance=1e-6  Setx0=off  InitialVoltage=0  Measurements=None
  i2_a : Outport
  i2_b : Outport  Port=2
  i2_c : Outport  Port=3
  vC_a : Outport  Port=4
  vC_b : Outport  Port=5
  vC_c : Outport  Port=6
  wires:
  up_a/1 -> Rate Transition13/1
  up_b/1 -> Rate Transition14/1
  up_c/1 -> Rate Transition15/1
  Rate Transition13/1 -> [up_a]
  Rate Transition14/1 -> [up_b]
  Rate Transition15/1 -> [up_c]
  Variação Paramétrica1/1 -> [p_ch]
  Inicialização/1 -> [init]
  Gain/1 -> PWM/1
  PWM/1 -> Conversor/1
  Mux/1 -> Gain/1
  [up_a] -> Controlled Voltage Source/1
  [up_b] -> Controlled Voltage Source1/1
  [up_c] -> Controlled Voltage Source2/1
  Multímetro/1 -> Demux/1
  Demux/1 -> i2_a/1
  Demux/2 -> i2_b/1
  Demux/3 -> i2_c/1
  Demux/4 -> vC_a/1
  Demux/5 -> vC_b/1
  Demux/6 -> vC_c/1
  [up_b] -> Mux/2
  [up_a] -> Mux/1
  [up_c] -> Mux/3
  Gain1/1 -> Ideal Switch4/1
  Gain2/1 -> Ideal Switch2/1
  Gain3/1 -> Ideal Switch/1
  [init] -> Ideal Switch6/1, Ideal Switch8/1, Ideal Switch7/1
  [p_ch] -> Gain1/1, Gain2/1, Gain3/1, Ideal Switch1/1, Ideal Switch3/1, Ideal Switch5/1
  connections:
  deltaL2a/RConn1 -- Ideal Switch8/LConn1 -- Rinit_a/LConn1 -- Ideal Switch/RConn1
  L1a/RConn1 -- Ca/LConn1 -- L2a+Lga/LConn1
  L2b+Lgb/LConn1 -- Cb/LConn1 -- L1b/RConn1
  L2c+Lgc/LConn1 -- Cc/LConn1 -- L1c/RConn1
  Ideal Switch/LConn1 -- L2a+Lga/RConn1 -- Ideal Switch1/LConn1
  Ideal Switch2/LConn1 -- L2b+Lgb/RConn1 -- Ideal Switch3/LConn1
  Ideal Switch4/LConn1 -- L2c+Lgc/RConn1 -- Ideal Switch5/LConn1
  Ca/RConn1 -- Cc/RConn1 -- Cb/RConn1
  Rinit_a/RConn1 -- Ideal Switch8/RConn1 -- Three-Phase Transformer (Two Windings)/LConn1
  Rinit_b/RConn1 -- Ideal Switch7/RConn1 -- Three-Phase Transformer (Two Windings)/LConn2
  Rinit_c/RConn1 -- Ideal Switch6/RConn1 -- Three-Phase Transformer (Two Windings)/LConn3
  deltaL2c/RConn1 -- Ideal Switch6/LConn1 -- Rinit_c/LConn1 -- Ideal Switch4/RConn1
  deltaL2b/RConn1 -- Ideal Switch7/LConn1 -- Rinit_b/LConn1 -- Ideal Switch2/RConn1
  Ground/LConn1 -- Controlled Voltage Source2/LConn1 -- Controlled Voltage Source1/LConn1 -- Controlled Voltage Source/LConn1
  Line 1 (300 km)/RConn2 -- Line 2 (300 km)/LConn2 -- Fault Breaker/LConn2
  Line 1 (300 km)/RConn1 -- Line 2 (300 km)/LConn1 -- Fault Breaker/LConn1
  Line 2 (300 km)/LConn3 -- Line 1 (300 km)/RConn3 -- Fault Breaker/LConn3
  Line 2 (300 km)/RConn1 -- B3/LConn1
  B3/LConn2 -- Line 2 (300 km)/RConn2
  L1b/LConn1 -- Controlled Voltage Source1/RConn1
  Controlled Voltage Source/RConn1 -- L1a/LConn1
  B3/RConn3 -- Three-Phase Source/RConn3
  Line 2 (300 km)/RConn3 -- B3/LConn3
  deltaL2b/LConn1 -- Ideal Switch3/RConn1
  L1c/LConn1 -- Controlled Voltage Source2/RConn1
  Conversor/RConn1 -- VCC/RConn1
  VCC/LConn1 -- Conversor/RConn2
  deltaL2a/LConn1 -- Ideal Switch1/RConn1
  deltaL2c/LConn1 -- Ideal Switch5/RConn1
  B3/RConn1 -- Three-Phase Source/RConn1
  B3/RConn2 -- Three-Phase Source/RConn2
